simulink library "csc_act_actuator_manager_lib"  (R2014b)
settings: Solver=ode45  StartTime=0.0  StopTime=10.0  RelTol=1e-3
undefined symbols (not defined in the file): est_time_step
libraries: csu_ftc_final_thruster_cmd_lib x1, util_info_lib x1, csu_taf_thruster_arm_fire_lib x1, csu_tcm_thruster_command_metering_lib x1
settings Model: Creator=ianmga  LastModifiedBy=mstewart

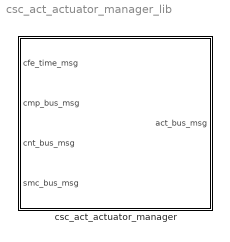
== system csc_act_actuator_manager_lib ==
  csc_act_actuator_manager : Subsystem  Tag=OFSW; MDL_TICK=CNT_BUS_MSG  TreatAsAtomicUnit=on  SystemSampleTime=est_time_step

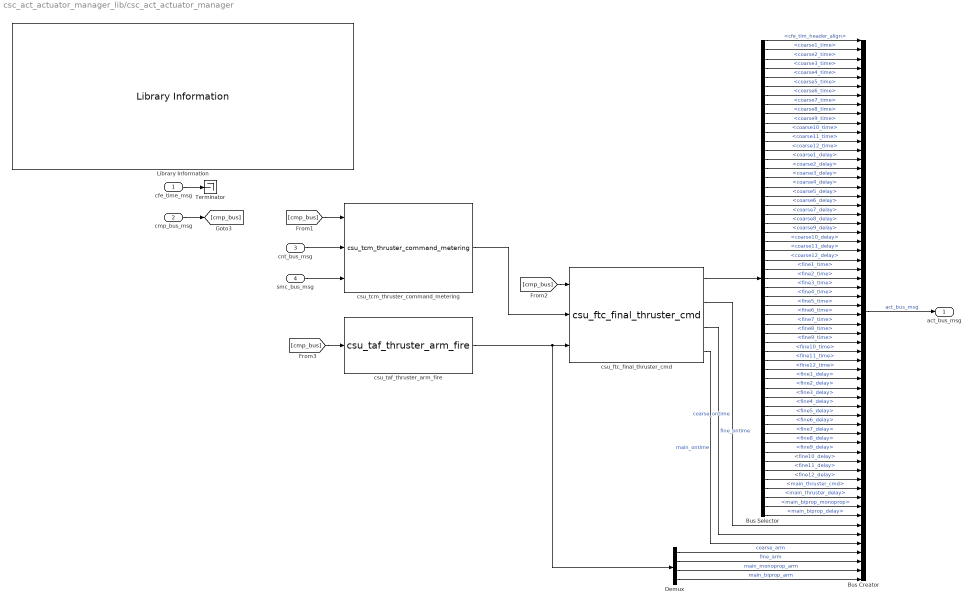
== system csc_act_actuator_manager_lib/csc_act_actuator_manager ==
  cfe_time_msg : Inport  OutDataTypeStr=Bus: cfe_time_msg
  cmp_bus_msg : Inport  Port=2
  cnt_bus_msg : Inport  Port=3  OutDataTypeStr=Bus: cnt_bus_msg
  smc_bus_msg : Inport  Port=4
  " csu_ftc_final_thruster_cmd" : csu_ftc_final_thruster_cmd_lib/ csu_ftc_final_thruster_cmd
  Bus Creator : BusCreator  Inputs=60  OutDataTypeStr=Bus: act_bus_msg  NonVirtualBus=on
  Bus Selector : BusSelector  OutputSignals=cfe_tlm_header_align,coarse1_time,coarse2_time,coarse3_time,coarse4_time,coarse5_time,coarse6_time,coarse7_time,coarse8_time,coarse9_time,coarse10_time,coarse11_time,coarse12_time,coarse1_delay,coarse2_delay,coarse3_delay,coarse4_delay,coarse5_delay,coarse6_delay,coarse7_delay,coarse8_delay,coarse9_delay,coarse10_delay,coarse11_delay,coarse12_delay,fine1_time,fine2_time,fine3_time,fine4_time,fine5_time,fine6_time,fine7_time,fine8_time,fine9_time,fine10_time,fine11_time,fine12_time,fine1_delay,fine2_delay,fine3_delay,fine4_delay,fine5_delay,fine6_delay,fine7_delay,fine8_delay,fine9_delay,fine10_delay,fine11_delay,fine12_delay,main_thruster_cmd,main_thruster_delay,main_biprop_monoprop,main_biprop_delay
  Demux : Demux  Outputs=[12 12 1 1]
  Library Information : util_info_lib/Library Information  owner='escrane'
  Terminator : Terminator
  csu_taf_thruster_arm_fire : csu_taf_thruster_arm_fire_lib/csu_taf_thruster_arm_fire
  csu_tcm_thruster_command_metering : csu_tcm_thruster_command_metering_lib/csu_tcm_thruster_command_metering
  act_bus_msg : Outport
  wires:
  Bus Creator/1 -> act_bus_msg/1  "act_bus_msg"
  [cmp_bus] -> csu_taf_thruster_arm_fire/1
  Demux/4 -> Bus Creator/60  "main_biprop_arm"
  Demux/3 -> Bus Creator/59  "main_monoprop_arm"
  Demux/2 -> Bus Creator/58  "fine_arm"
  Demux/1 -> Bus Creator/57  "coarse_arm"
  " csu_ftc_final_thruster_cmd"/4 -> Bus Creator/56  "main_ontime"
  " csu_ftc_final_thruster_cmd"/3 -> Bus Creator/55  "fine_ontime"
  " csu_ftc_final_thruster_cmd"/2 -> Bus Creator/54  "coarse_ontime"
  " csu_ftc_final_thruster_cmd"/1 -> Bus Selector/1
  Bus Selector/7 -> Bus Creator/7  "<coarse6_time>"
  Bus Selector/20 -> Bus Creator/20  "<coarse7_delay>"
  Bus Selector/35 -> Bus Creator/35  "<fine10_time>"
  Bus Selector/31 -> Bus Creator/31  "<fine6_time>"
  Bus Selector/48 -> Bus Creator/48  "<fine11_delay>"
  Bus Selector/18 -> Bus Creator/18  "<coarse5_delay>"
  Bus Selector/42 -> Bus Creator/42  "<fine5_delay>"
  Bus Selector/30 -> Bus Creator/30  "<fine5_time>"
  Bus Selector/28 -> Bus Creator/28  "<fine3_time>"
  Bus Selector/4 -> Bus Creator/4  "<coarse3_time>"
  Bus Selector/37 -> Bus Creator/37  "<fine12_time>"
  Bus Selector/33 -> Bus Creator/33  "<fine8_time>"
  Bus Selector/40 -> Bus Creator/40  "<fine3_delay>"
  Bus Selector/13 -> Bus Creator/13  "<coarse12_time>"
  Bus Selector/10 -> Bus Creator/10  "<coarse9_time>"
  Bus Selector/23 -> Bus Creator/23  "<coarse10_delay>"
  Bus Selector/53 -> Bus Creator/53  "<main_biprop_delay>"
  Bus Selector/24 -> Bus Creator/24  "<coarse11_delay>"
  Bus Selector/16 -> Bus Creator/16  "<coarse3_delay>"
  Bus Selector/41 -> Bus Creator/41  "<fine4_delay>"
  Bus Selector/50 -> Bus Creator/50  "<main_thruster_cmd>"
  Bus Selector/49 -> Bus Creator/49  "<fine12_delay>"
  Bus Selector/45 -> Bus Creator/45  "<fine8_delay>"
  Bus Selector/43 -> Bus Creator/43  "<fine6_delay>"
  Bus Selector/44 -> Bus Creator/44  "<fine7_delay>"
  Bus Selector/14 -> Bus Creator/14  "<coarse1_delay>"
  Bus Selector/29 -> Bus Creator/29  "<fine4_time>"
  Bus Selector/19 -> Bus Creator/19  "<coarse6_delay>"
  Bus Selector/17 -> Bus Creator/17  "<coarse4_delay>"
  Bus Selector/38 -> Bus Creator/38  "<fine1_delay>"
  Bus Selector/9 -> Bus Creator/9  "<coarse8_time>"
  Bus Selector/3 -> Bus Creator/3  "<coarse2_time>"
  Bus Selector/5 -> Bus Creator/5  "<coarse4_time>"
  Bus Selector/6 -> Bus Creator/6  "<coarse5_time>"
  Bus Selector/51 -> Bus Creator/51  "<main_thruster_delay>"
  Bus Selector/27 -> Bus Creator/27  "<fine2_time>"
  Bus Selector/32 -> Bus Creator/32  "<fine7_time>"
  Bus Selector/52 -> Bus Creator/52  "<main_biprop_monoprop>"
  Bus Selector/21 -> Bus Creator/21  "<coarse8_delay>"
  Bus Selector/26 -> Bus Creator/26  "<fine1_time>"
  Bus Selector/8 -> Bus Creator/8  "<coarse7_time>"
  Bus Selector/47 -> Bus Creator/47  "<fine10_delay>"
  Bus Selector/15 -> Bus Creator/15  "<coarse2_delay>"
  Bus Selector/39 -> Bus Creator/39  "<fine2_delay>"
  Bus Selector/34 -> Bus Creator/34  "<fine9_time>"
  Bus Selector/25 -> Bus Creator/25  "<coarse12_delay>"
  Bus Selector/11 -> Bus Creator/11  "<coarse10_time>"
  Bus Selector/46 -> Bus Creator/46  "<fine9_delay>"
  Bus Selector/12 -> Bus Creator/12  "<coarse11_time>"
  Bus Selector/22 -> Bus Creator/22  "<coarse9_delay>"
  Bus Selector/36 -> Bus Creator/36  "<fine11_time>"
  Bus Selector/2 -> Bus Creator/2  "<coarse1_time>"
  Bus Selector/1 -> Bus Creator/1  "<cfe_tlm_header_align>"
  cfe_time_msg/1 -> Terminator/1
  csu_tcm_thruster_command_metering/1 -> " csu_ftc_final_thruster_cmd"/2
  csu_taf_thruster_arm_fire/1 -> " csu_ftc_final_thruster_cmd"/3, Demux/1
  cmp_bus_msg/1 -> [cmp_bus]
  [cmp_bus] -> csu_tcm_thruster_command_metering/1
  [cmp_bus] -> " csu_ftc_final_thruster_cmd"/1
  cnt_bus_msg/1 -> csu_tcm_thruster_command_metering/2
  smc_bus_msg/1 -> csu_tcm_thruster_command_metering/3
